simulink model "hyd_hyb_2_int_cont_Final_AMT"  (R2013b)
settings: Solver=ode4  StartTime=0  StopTime=3005  FixedStep=0.01  MaxStep=.4  RelTol=1e-8
InitFcn:
  | const_3_new
values from neighbouring files (symbols this model uses):
  Af = 6.3    [brk_enrg.m]    (also in brk_enrg_1.m)
  BSFC_906_205 = [3.5684 4.3466 5.1668 6.0769 6.988 7.8992 8.8104 9.7336 10.8548 11.9809 13.1112 14.2571 ... (663 elements, 39x17)]    [BSFC_map_906_205.mat]
  Cd = 0.55    [brk_enrg.m]    (also in brk_enrg_1.m)
  den = 1.202    [brk_enrg.m]    (also in brk_enrg_1.m)
  fr = 0.01    [brk_enrg.m]    (also in brk_enrg_1.m)
undefined symbols (not defined in the file or in its folder): clutchRise, down_spd_2, down_spd_3, down_spd_4, down_spd_c, Driving_Cycle, fuel_density, gearshift, I_wheel, Idle_spd_eng_906, M1_hydr, p_v_15, pmax_125, qv_125, Rw, sec_eng_sfc_map, T0, T1, T_max_906, T_min, TC_spd_ratio_max, teta_new_10, torque_convertor, Twait, up_spd_1, up_spd_2, up_spd_3, up_spd_c, v_p_10, v_p_15, v_p_5
libraries: neural x1742, fl_lib x43, nesl_utility x30, sdl_lib x14, simulink x4, simulink_need_slupdate x1
(part 16 of 26)

== system hyd_hyb_2_int_cont_Final_AMT/controller1/optimized controller/SOC upper 0.5/SOC upper 0.6/SOC under 0.7/net_col_e_f_6_7/Layer 3/LW{3,2} ==
  "ad{3,2}" : Inport  PortDimensions=50
  "IW{3,2}(1,:)'" : Constant  Value=[-0.14496716486052699;-0.47354696627688647;0.54035576647762795;-0.68602701998320026;0.46484597614576872;0.47734251614963863;-0.60562651050231653;-0.98169339990592763;-0.30180585453035474;-1.044123812618281;0.3636963831357668;-0.2721056979576707;-0.62844162818310545;0.94114408156053864;0.032914194045848055;-0.70828972200722162;-0.82926105695241381;1.0228798230235354;0.14407210144155363;1.0151191535640738;-0.23736565494839279;0.77950027844319802;0.5516930677089682;0.54397813376888204;-0.83798239366063099;-0.018703325160830467;0.89876421382365645;-0.18305519296728018;-0.86198808218664358;-0.52658495578222264;0.45074819920239834;0.88005946883701902;-0.66967180109277658;-0.9152247806304189;0.52672733175493625;0.10197970386169893;0.46507499018683973;0.28571426570795944;-0.42251150852828617;1.0351916215442039;0.73732399198222975;0.43774975692502838;0.70933394438012298;-0.32202855182503765;-0.0051672403457150989;-0.53858112522985413;0.24285543394581888;0.44661184140456672;0.45838623581582921;-0.94350953461835607]
  Mux : Mux  Inputs=1
  dotprod1 : neural/Weight Functions/dotprod
  "lz{3,2}" : Outport
  wires:
  Mux/1 -> "lz{3,2}"/1
  dotprod1/1 -> Mux/1
  "ad{3,2}"/1 -> dotprod1/2
  "IW{3,2}(1,:)'"/1 -> dotprod1/1

== system hyd_hyb_2_int_cont_Final_AMT/controller1/optimized controller/SOC upper 0.5/SOC upper 0.6/SOC under 0.7/net_loc_rod_6_7/Layer 1/Delays 1 ==
  "p{1}" : Inport  PortDimensions=2
  mux : Mux  Inputs=1
  "pd{1,1}" : Outport
  wires:
  mux/1 -> "pd{1,1}"/1
  "p{1}"/1 -> mux/1

== system hyd_hyb_2_int_cont_Final_AMT/controller1/optimized controller/SOC upper 0.5/SOC upper 0.6/SOC under 0.7/net_loc_rod_6_7/Layer 1/IW{1,1} ==
  "pd{1,1}" : Inport  PortDimensions=2
  "IW{1,1}(1,:)'" : Constant  Value=[-7.2537115098885474;5.1245030557382769]
  "IW{1,1}(10,:)'" : Constant  Value=[-8.5591399578865293;2.2634745296375076]
  "IW{1,1}(11,:)'" : Constant  Value=[8.7835694285365591;1.2801494147307597]
  "IW{1,1}(12,:)'" : Constant  Value=[7.8321129027526517;-4.1878865124292659]
  "IW{1,1}(13,:)'" : Constant  Value=[8.5750438304460825;-2.2136685825202154]
  "IW{1,1}(14,:)'" : Constant  Value=[4.5041422704461889;7.6277220573690911]
  "IW{1,1}(15,:)'" : Constant  Value=[2.4040741087696262;-8.5404453945895806]
  "IW{1,1}(16,:)'" : Constant  Value=[-2.1668409405480351;-8.600460377144687]
  "IW{1,1}(17,:)'" : Constant  Value=[8.3353033855566121;-3.030430277914419]
  "IW{1,1}(18,:)'" : Constant  Value=[5.0945559135427825;7.2508738408169346]
  "IW{1,1}(19,:)'" : Constant  Value=[-8.8509907019625906;-0.21982707435322274]
  "IW{1,1}(2,:)'" : Constant  Value=[4.5739747394442629;-7.6315572401942058]
  "IW{1,1}(20,:)'" : Constant  Value=[3.6600253756129688;-8.0597703880573217]
  "IW{1,1}(21,:)'" : Constant  Value=[7.8850321171524431;-4.0224485296002372]
  "IW{1,1}(22,:)'" : Constant  Value=[-7.3670984282951641;-4.9167356657284644]
  "IW{1,1}(23,:)'" : Constant  Value=[-8.4520982729402494;2.6506135219515903]
  "IW{1,1}(24,:)'" : Constant  Value=[4.2649597192404602;-7.7628029668267153]
  "IW{1,1}(25,:)'" : Constant  Value=[-2.6533017882247014;-8.452799924104804]
  "IW{1,1}(26,:)'" : Constant  Value=[-8.6342242991695475;-2.0851850503255651]
  "IW{1,1}(27,:)'" : Constant  Value=[2.8571555118263285;8.3799699643561318]
  "IW{1,1}(28,:)'" : Constant  Value=[-5.8585035631892382;-6.6167886360787511]
  "IW{1,1}(29,:)'" : Constant  Value=[5.549840815037097;6.941726895804802]
  "IW{1,1}(3,:)'" : Constant  Value=[-8.8674383725969967;-0.49348374013382512]
  "IW{1,1}(30,:)'" : Constant  Value=[7.5317845772137666;-4.9212498919710939]
  "IW{1,1}(31,:)'" : Constant  Value=[-8.8371653005134583;1.1147497029752584]
  "IW{1,1}(32,:)'" : Constant  Value=[-5.555189944475508;-6.9308932773263985]
  "IW{1,1}(33,:)'" : Constant  Value=[4.1366694932745984;7.8303800993524373]
  "IW{1,1}(34,:)'" : Constant  Value=[-4.4192059733022022;-7.6664850452561604]
  "IW{1,1}(35,:)'" : Constant  Value=[6.2012468696204115;6.4066347869806242]
  "IW{1,1}(36,:)'" : Constant  Value=[-2.9731271609116319;-8.3658880105352527]
  "IW{1,1}(37,:)'" : Constant  Value=[-8.4189097713904637;2.9674629023892365]
  "IW{1,1}(38,:)'" : Constant  Value=[8.3550511045513911;-3.1889153294931329]
  "IW{1,1}(39,:)'" : Constant  Value=[-5.5401688708317733;-7.0482233474690075]
  "IW{1,1}(4,:)'" : Constant  Value=[-4.0344896449520018;-7.8869017607918428]
  "IW{1,1}(40,:)'" : Constant  Value=[8.0122109115600377;-3.9438583373413363]
  "IW{1,1}(5,:)'" : Constant  Value=[-4.1359429686776901;-7.8358807582871748]
  "IW{1,1}(6,:)'" : Constant  Value=[5.6875032885297339;6.8518843981758728]
  "IW{1,1}(7,:)'" : Constant  Value=[4.4956619097616644;-7.7258116517018589]
  "IW{1,1}(8,:)'" : Constant  Value=[7.2546236624407117;5.0753363371884808]
  "IW{1,1}(9,:)'" : Constant  Value=[-0.81542568460144016;8.8325278289838707]
  Mux : Mux  Inputs=40
  dotprod{1..40} (40 alike) : neural/Weight Functions/dotprod
  "iz{1,1}" : Outport
  wires:
  Mux/1 -> "iz{1,1}"/1
  dotprod40/1 -> Mux/40
  "IW{1,1}(40,:)'"/1 -> dotprod40/1
  dotprod39/1 -> Mux/39
  "IW{1,1}(39,:)'"/1 -> dotprod39/1
  dotprod38/1 -> Mux/38
  "IW{1,1}(38,:)'"/1 -> dotprod38/1
  dotprod37/1 -> Mux/37
  "IW{1,1}(37,:)'"/1 -> dotprod37/1
  dotprod36/1 -> Mux/36
  "IW{1,1}(36,:)'"/1 -> dotprod36/1
  dotprod35/1 -> Mux/35
  "IW{1,1}(35,:)'"/1 -> dotprod35/1
  dotprod34/1 -> Mux/34
  "IW{1,1}(34,:)'"/1 -> dotprod34/1
  dotprod33/1 -> Mux/33
  "IW{1,1}(33,:)'"/1 -> dotprod33/1
  dotprod32/1 -> Mux/32
  "IW{1,1}(32,:)'"/1 -> dotprod32/1
  dotprod31/1 -> Mux/31
  "IW{1,1}(31,:)'"/1 -> dotprod31/1
  dotprod30/1 -> Mux/30
  "IW{1,1}(30,:)'"/1 -> dotprod30/1
  dotprod29/1 -> Mux/29
  "IW{1,1}(29,:)'"/1 -> dotprod29/1
  dotprod28/1 -> Mux/28
  "IW{1,1}(28,:)'"/1 -> dotprod28/1
  dotprod27/1 -> Mux/27
  "IW{1,1}(27,:)'"/1 -> dotprod27/1
  dotprod26/1 -> Mux/26
  "IW{1,1}(26,:)'"/1 -> dotprod26/1
  dotprod25/1 -> Mux/25
  "IW{1,1}(25,:)'"/1 -> dotprod25/1
  dotprod24/1 -> Mux/24
  "IW{1,1}(24,:)'"/1 -> dotprod24/1
  dotprod23/1 -> Mux/23
  "IW{1,1}(23,:)'"/1 -> dotprod23/1
  dotprod22/1 -> Mux/22
  "IW{1,1}(22,:)'"/1 -> dotprod22/1
  dotprod21/1 -> Mux/21
  "IW{1,1}(21,:)'"/1 -> dotprod21/1
  dotprod20/1 -> Mux/20
  "IW{1,1}(20,:)'"/1 -> dotprod20/1
  dotprod19/1 -> Mux/19
  "IW{1,1}(19,:)'"/1 -> dotprod19/1
  dotprod18/1 -> Mux/18
  "IW{1,1}(18,:)'"/1 -> dotprod18/1
  dotprod17/1 -> Mux/17
  "IW{1,1}(17,:)'"/1 -> dotprod17/1
  dotprod16/1 -> Mux/16
  "IW{1,1}(16,:)'"/1 -> dotprod16/1
  dotprod15/1 -> Mux/15
  "IW{1,1}(15,:)'"/1 -> dotprod15/1
  dotprod14/1 -> Mux/14
  "IW{1,1}(14,:)'"/1 -> dotprod14/1
  dotprod13/1 -> Mux/13
  "IW{1,1}(13,:)'"/1 -> dotprod13/1
  dotprod12/1 -> Mux/12
  "IW{1,1}(12,:)'"/1 -> dotprod12/1
  dotprod11/1 -> Mux/11
  "IW{1,1}(11,:)'"/1 -> dotprod11/1
  dotprod10/1 -> Mux/10
  "IW{1,1}(10,:)'"/1 -> dotprod10/1
  dotprod9/1 -> Mux/9
  "IW{1,1}(9,:)'"/1 -> dotprod9/1
  dotprod8/1 -> Mux/8
  "IW{1,1}(8,:)'"/1 -> dotprod8/1
  dotprod7/1 -> Mux/7
  "IW{1,1}(7,:)'"/1 -> dotprod7/1
  dotprod6/1 -> Mux/6
  "IW{1,1}(6,:)'"/1 -> dotprod6/1
  dotprod5/1 -> Mux/5
  "IW{1,1}(5,:)'"/1 -> dotprod5/1
  dotprod4/1 -> Mux/4
  "IW{1,1}(4,:)'"/1 -> dotprod4/1
  dotprod3/1 -> Mux/3
  "IW{1,1}(3,:)'"/1 -> dotprod3/1
  dotprod2/1 -> Mux/2
  "IW{1,1}(2,:)'"/1 -> dotprod2/1
  dotprod1/1 -> Mux/1
  "pd{1,1}"/1 -> dotprod40/2, dotprod39/2, dotprod38/2, dotprod37/2, dotprod36/2, dotprod35/2, dotprod34/2, dotprod33/2, dotprod32/2, dotprod31/2, dotprod30/2, dotprod29/2, dotprod28/2, dotprod27/2, dotprod26/2, dotprod25/2, dotprod24/2, dotprod23/2, dotprod22/2, dotprod21/2, dotprod20/2, dotprod19/2, dotprod18/2, dotprod17/2, dotprod16/2, dotprod15/2, dotprod14/2, dotprod13/2, dotprod12/2, dotprod11/2, dotprod10/2, dotprod9/2, dotprod8/2, dotprod7/2, dotprod6/2, dotprod5/2, dotprod4/2, dotprod3/2, dotprod2/2, dotprod1/2
  "IW{1,1}(1,:)'"/1 -> dotprod1/1

== system hyd_hyb_2_int_cont_Final_AMT/controller1/optimized controller/SOC upper 0.5/SOC upper 0.6/SOC under 0.7/net_loc_rod_6_7/Layer 2/Delays 1 ==
  "p{2}" : Inport  PortDimensions=40
  mux : Mux  Inputs=1
  "pd{2,1}" : Outport
  wires:
  mux/1 -> "pd{2,1}"/1
  "p{2}"/1 -> mux/1
